simulink model "SineWave_Combination_Example"  (R2014a)
settings: Solver=ode3  StartTime=0.0  StopTime=3e-3  FixedStep=1e-5  RelTol=1e-3
settings Model: Creator=Lee  LastModifiedBy=Lee
settings DataIOCC: SignalLoggingSaveFormat=ModelDataLogs
settings OptimizationCC: ExpressionDepthLimit=2147483647
settings DebuggingCC: UnderspecifiedInitializationDetection=Classic  SolverPrmCheckMsg=none  FcnCallInpInsideContextMsg=UseLocalSettings  StateNameClashWarn=warning
settings GRTTargetCC: CombineOutputUpdateFcns=off  GRTInterface=on

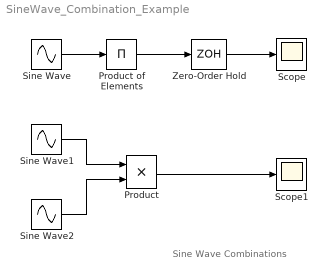
== system SineWave_Combination_Example ==
  note: Sine Wave Combinations
  Product : Product  RndMeth=Zero
  Product of Elements : Product  Inputs=*
  Scope : Scope
  Scope1 : Scope
  Sine Wave : Sin  Amplitude=[2 1]  Bias=[0 1]  Frequency=2*pi*[10 1]*1e3  SampleTime=0
  Sine Wave1 : Sin  Bias=2  Frequency=2*pi*1e3  SampleTime=0
  Sine Wave2 : Sin  Frequency=2*pi*10e3  SampleTime=0
  Zero-Order Hold : ZeroOrderHold  SampleTime=2e-5
  wires:
  Sine Wave/1 -> Product of Elements/1
  Product of Elements/1 -> Zero-Order Hold/1
  Zero-Order Hold/1 -> Scope/1
  Sine Wave1/1 -> Product/1
  Sine Wave2/1 -> Product/2
  Product/1 -> Scope1/1
